simulink model "CTRL_SPECCTRL_FB_STRAT3_test"  (R2024b)
settings: Solver=VariableStepAuto  StartTime=0.0  StopTime=10.0  RelTol=1e-3
libraries: CTRL_SPECCTRL_FB_STRAT3 x1
settings Model: Creator=blatak  LastModifiedBy=blatak

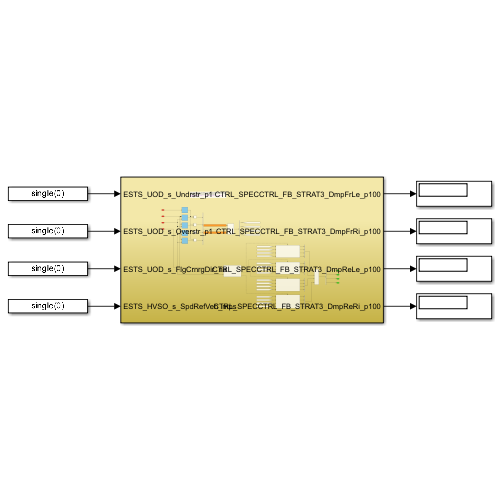
[thumbnail: Simulink's stored preview of the top-level diagram]
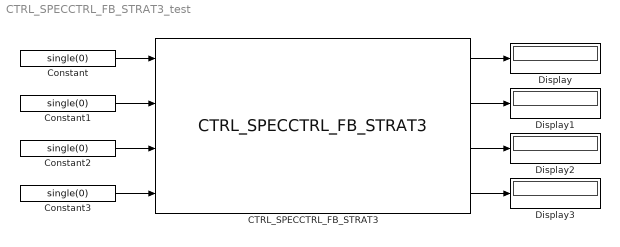
== system CTRL_SPECCTRL_FB_STRAT3_test ==
  CTRL_SPECCTRL_FB_STRAT3 : CTRL_SPECCTRL_FB_STRAT3/CTRL_SPECCTRL_FB_STRAT3  SystemSampleTime=-1  VariantActivationTime=update diagram  AllowFlexibleInterface=on  Latency=0  AutoFrameSizeCalculation=off
  Constant{,1..3} (4 alike) : Constant  Value=single(0)
  Display{,1..3} (4 alike) : Display
  wires:
  Constant/1 -> CTRL_SPECCTRL_FB_STRAT3/1
  Constant1/1 -> CTRL_SPECCTRL_FB_STRAT3/2
  Constant2/1 -> CTRL_SPECCTRL_FB_STRAT3/3
  Constant3/1 -> CTRL_SPECCTRL_FB_STRAT3/4
  CTRL_SPECCTRL_FB_STRAT3/1 -> Display/1
  CTRL_SPECCTRL_FB_STRAT3/2 -> Display1/1
  CTRL_SPECCTRL_FB_STRAT3/3 -> Display2/1
  CTRL_SPECCTRL_FB_STRAT3/4 -> Display3/1
